simulink model "CountOvf_step4"  (R2014b)
settings: Solver=FixedStepDiscrete  SolverMode=SingleTasking  StartTime=0.0  StopTime=1000  RelTol=1e-3
libraries: simulink x1, hdlsllib x1
settings Model: Creator=amatsumo  LastModifiedBy=kotsuka
settings DataIOCC: SignalLoggingSaveFormat=ModelDataLogs  SaveOutput=off  SignalLogging=off  SaveTime=off
settings OptimizationCC: BlockReduction=off  ConditionallyExecuteInputs=off  InlineParams=on  ExpressionDepthLimit=2147483647
settings DebuggingCC: AlgebraicLoopMsg=error  UnderspecifiedInitializationDetection=Classic  MergeDetectMultiDrivingBlocksExec=none  SingleTaskRateTransMsg=error  FcnCallInpInsideContextMsg=UseLocalSettings  StateNameClashWarn=warning
settings HardwareCC: ProdHWDeviceType=ASIC/FPGA->ASIC/FPGA  ProdEqTarget=off
settings SFSimCC: SimParseCustomCode=off
settings GRTTargetCC: CombineOutputUpdateFcns=off  GRTInterface=on

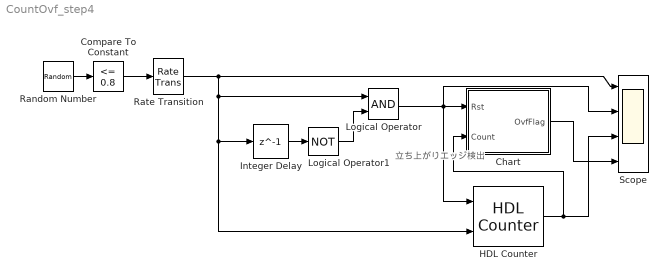
== system CountOvf_step4 ==
  note: 立ち上がりエッジ検出
  Chart : Stateflow chart  TreatAsAtomicUnit=on
  Compare To Constant : simulink/Logic and Bit Operations/Compare To Constant  relop=<=  const=0.8  OutDataTypeStr=boolean  ZeroCross=off
  HDL Counter : hdlsllib/HDL Operations/HDL Counter  CountType=Free running  CountInit=1  CountStep=1  CountMax=100  CountFromType=Initial value  CountFrom=1  CountResetPort=on  CountLoadPort=off  CountEnbPort=on  CountDirPort=off  CountDataType=Unsigned  CountWordLen=8  CountFracLen=0  CountSampTime=1
  Integer Delay : Delay  DelayLength=1  InputProcessing=Inherited
  Logical Operator : Logic  AllPortsSameDT=off  OutDataTypeStr=boolean
  Logical Operator1 : Logic  Operator=NOT  AllPortsSameDT=off  OutDataTypeStr=boolean
  Random Number : RandomNumber  SampleTime=70
  Rate Transition : RateTransition  OutPortSampleTime=1
  Scope : Scope  NumInputPorts=4
      settings: TimeRange=1000  YMin=-1~-1~-1~-5  YMax=2~2~260~5
  wires:
  HDL Counter/1 -> Chart/2(Count), Scope/3
  Rate Transition/1 -> Logical Operator/1, Integer Delay/1, HDL Counter/2, Scope/1
  Integer Delay/1 -> Logical Operator1/1
  Logical Operator1/1 -> Logical Operator/2
  Random Number/1 -> Compare To Constant/1
  Compare To Constant/1 -> Rate Transition/1
  Logical Operator/1 -> HDL Counter/1, Chart/1(Rst), Scope/2
  Chart/1(OvfFlag) -> Scope/4

== stateflow chart CountOvf_step4/Chart ==
  settings: stateMachineType=MEALY_MACHINE  executeAtInitialization=1  initializeOutput=1
  state CountMax
  state Init
  state Ovf
  (default) -> Init
  Init -> CountMax [order 1] : [Count >= 255]
      | {OvfFlag = 0;}
  Init -> Init [order 2] : {OvfFlag = 0;}
  CountMax -> Init [order 2] : {OvfFlag = 0;}
  Ovf -> Init [order 1] : [Rst == 1]
      | {OvfFlag = 0;}
  CountMax -> Ovf [order 1] : [Count == 0]
      | {OvfFlag = 1;}
  Ovf -> Ovf [order 2] : {OvfFlag = 1;}
  data: Rst input boolean; OvfFlag output boolean; Count input uint8
